simulink model "eme185"  (Simulink 8.6)
settings: Solver=VariableStepAuto  StartTime=0.0  StopTime=10  RelTol=1e-3
values from neighbouring files (symbols this model uses):
  a = [(-2/tau - 1/tau_0) 1/tau 1/tau; 1/tau -2/tau 1/tau; 1/tau 1/tau -2/tau]    [MAE_272A_HW2_Q1a.m]    (also in Vehicle_Dynamic_main.m = 0.624; Vehicle_Dynamic_main_V0.m = 0.624; Vehicle_Dynamic_main_V01.m = 0.624; Vehicle_Dynamic_main_V0605.m = 0.624)
  b = [1/A 0; 0 1/A; 0 0]    [MAE_272A_HW2_Q1a.m]    (also in Vehicle_Dynamic_main.m = 0.624; Vehicle_Dynamic_main_V0.m = 0.624; Vehicle_Dynamic_main_V01.m = 0.624; Vehicle_Dynamic_main_V0605.m = 0.624)
  bL = 60    [simulation_1.m]
  bm = 0.005    [simulation_1.m]
  Ca = 1*0.025    (= 0.025)    [simulation_1.m]
  Cy = 2*20000    (= 40000)    [simulation_1.m]
  gr = 1/20    (= 0.05)    [simulation_1.m]
  initial = [0 0 0 0 (m*g*weight_left/k_spring) (m*g*weight_right/k_spring) ((m*weight_left+mt)*g/k_tire_l) ((m*weight_right+mt)*g/k_tire_r) 0]    [Wegiht_Transfer_Calculator.m]    (also in simulation_1.m = [0 0 0 0 0 0 0 0 0 0])
  Jm = 3.5e-4    (= 0.00035)    [simulation_1.m]
  Jwd = 0.45    [simulation_1.m]
  Jy = 0.4*m*a*b    (= 864)    [master.m]    (also in simulation_1.m = 4250)
  kL = 1400    [simulation_1.m]
  kU = 140    [simulation_1.m]
  l = 0.135    [simulation_1.m]
  m = m_total*weight_front    (= 118.8)    [Wegiht_Transfer_Calculator.m]    (also in master.m = 1600; simulation_1.m = 1800)
  rp = 0.01    [simulation_1.m]
  T = minreal(1-S)    [MAE298_Final_Q2.m]    (also in MAE298_Final_Q22.m = 1-S; MAE298_Final_Q5.m = zpk(minreal(Y*Gp)); MAE_s72A_HW4_Q4.m = 1-S; MAE_s72A_HW4_Q4_5.m = 1-S)
settings Model: Creator=zzLiu  LastModifiedBy=zzLiu
settings DataIOCC: SaveFormat=Dataset  SignalLoggingSaveFormat=Dataset
settings OptimizationCC: ExpressionDepthLimit=128
settings DebuggingCC: UnderspecifiedInitializationDetection=Simplified  MergeDetectMultiDrivingBlocksExec=error  SolverPrmCheckMsg=none  FcnCallInpInsideContextMsg=EnableAllAsError  StateNameClashWarn=none
settings HardwareCC: ProdBitPerPointer=64  ProdLargestAtomicFloat=Float  ProdIntDivRoundTo=Zero  ProdEndianess=LittleEndian  ProdWordSize=64  ProdHWDeviceType=Intel->x86-64 (Windows64)
settings GRTTargetCC: GeneratePreprocessorConditionals=Use local settings  CombineOutputUpdateFcns=on  GRTInterface=off
settings ConfigComp: CovModelRefEnable=off

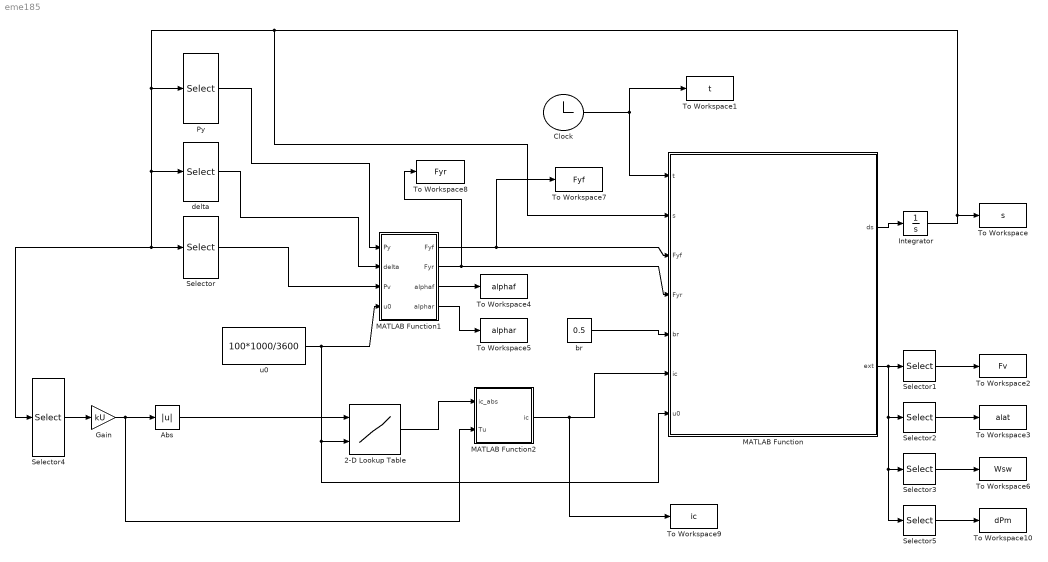
== system eme185 ==
  2-D Lookup Table : Lookup_n-D  BreakpointsForDimension1=[0.0 0.6 1.1 1.6 2.1 2.6 3.2 3.7 4.2 4.7 5.2 5.7 6.3]  BreakpointsForDimension2=[0 5.5556 11.1111 22.2222 27.7778 33.3333]  Table=[0 0 0 1.1 2.0 7.0 14.6 22.3 29.7 37.4 45.0 45.0 45.0;0 0 0 0 0 5.4 12.6 19.1 25.0 31.1 36.5 40.5 40.5;0 0 0 0 0 4.7 10.6 16.4 21.6 27.2 32.4 36.0 36.0;0 0 0 0.5 1.5 4.1 7.7 11.5 15.8 19.8 23.0 23.0 23.0;0 0 0 0 0 2.9 6.1 9.5 12.8 16.7 22.1 22.1 22.1;0 0 0 0 0 2.3 5.0 7.9 11.7 15.1 22.1 22.1 22.1]'  InternalRulePriority=Speed  RndMeth=Simplest  InputSameDT=on
  Abs : Abs
  Clock : Clock
  Gain : Gain  Gain=kU
  Integrator : Integrator  InitialCondition=initial
  MATLAB Function : MATLAB Function  TreatAsAtomicUnit=on
  MATLAB Function1 : MATLAB Function  TreatAsAtomicUnit=on
  MATLAB Function2 : MATLAB Function  TreatAsAtomicUnit=on
  Py : Selector  InputPortWidth=10  IndexOptions=Index vector (dialog)  Indices=[2]  OutputSizes=1
  Selector : Selector  InputPortWidth=10  IndexOptions=Index vector (dialog)  Indices=[1]  OutputSizes=1
  Selector1 : Selector  InputPortWidth=4  IndexOptions=Index vector (dialog)  Indices=[1]  OutputSizes=1
  Selector2 : Selector  InputPortWidth=4  IndexOptions=Index vector (dialog)  Indices=[2]  OutputSizes=1
  Selector3 : Selector  InputPortWidth=4  IndexOptions=Index vector (dialog)  Indices=[3]  OutputSizes=1
  Selector4 : Selector  InputPortWidth=10  IndexOptions=Index vector (dialog)  Indices=[5]  OutputSizes=1
  Selector5 : Selector  InputPortWidth=4  IndexOptions=Index vector (dialog)  Indices=[4]  OutputSizes=1
  To Workspace : ToWorkspace  VariableName=s  SampleTime=-1
  To Workspace1 : ToWorkspace  VariableName=t  SampleTime=-1
  To Workspace10 : ToWorkspace  VariableName=dPm  SaveFormat=Timeseries  SampleTime=-1
  To Workspace2 : ToWorkspace  VariableName=Fv  SaveFormat=Timeseries  SampleTime=-1
  To Workspace3 : ToWorkspace  VariableName=alat  SaveFormat=Timeseries  SampleTime=-1
  To Workspace4 : ToWorkspace  VariableName=alphaf  SaveFormat=Timeseries  SampleTime=-1
  To Workspace5 : ToWorkspace  VariableName=alphar  SaveFormat=Timeseries  SampleTime=-1
  To Workspace6 : ToWorkspace  VariableName=Wsw  SaveFormat=Timeseries  SampleTime=-1
  To Workspace7 : ToWorkspace  VariableName=Fyf  SaveFormat=Timeseries  SampleTime=-1
  To Workspace8 : ToWorkspace  VariableName=Fyr  SaveFormat=Timeseries  SampleTime=-1
  To Workspace9 : ToWorkspace  VariableName=ic  SaveFormat=Timeseries  SampleTime=-1
  br : Constant  Value=0.5
  delta : Selector  InputPortWidth=10  IndexOptions=Index vector (dialog)  Indices=[7]  OutputSizes=1
  u0 : Constant  Value=100*1000/3600
  wires:
  MATLAB Function/1(ds) -> Integrator/1
  Integrator/1 -> MATLAB Function/2(s), Selector/1, Selector4/1, delta/1, Py/1, To Workspace/1
  br/1 -> MATLAB Function/5(br)
  MATLAB Function1/1(Fyf) -> To Workspace7/1, MATLAB Function/3(Fyf)
  MATLAB Function1/2(Fyr) -> MATLAB Function/4(Fyr), To Workspace8/1
  Py/1 -> MATLAB Function1/1(Py)
  delta/1 -> MATLAB Function1/2(delta)
  Clock/1 -> To Workspace1/1, MATLAB Function/1(t)
  u0/1 -> MATLAB Function/7(u0), 2-D Lookup Table/2, MATLAB Function1/4(u0)
  Selector/1 -> MATLAB Function1/3(Pv)
  MATLAB Function1/3(alphaf) -> To Workspace4/1
  MATLAB Function1/4(alphar) -> To Workspace5/1
  MATLAB Function/2(ext) -> Selector5/1, Selector3/1, Selector2/1, Selector1/1
  Selector1/1 -> To Workspace2/1
  Selector2/1 -> To Workspace3/1
  Selector3/1 -> To Workspace6/1
  Selector4/1 -> Gain/1
  Gain/1 -> MATLAB Function2/2(Tu), Abs/1
  Selector5/1 -> To Workspace10/1
  Abs/1 -> 2-D Lookup Table/1
  2-D Lookup Table/1 -> MATLAB Function2/1(ic_abs)
  MATLAB Function2/1(ic) -> To Workspace9/1, MATLAB Function/6(ic)

== matlab function MATLAB Function1 ==
  data: Py input double; Fyf output double; delta input double; a parameter double; b parameter double; Cy parameter double; Jy parameter double; m parameter double; Pv input double; u0 input double; Fyr output double; alphaf output double; alphar output double
function [Fyf,Fyr,alphaf,alphar] = fcn(Py, delta, a, b, Cy,Jy, m, Pv,u0)
%#codegen

wy = Py/Jy;
v = Pv/m;

alphaf = delta - atan((v+a*wy)/u0);
alphar = -atan((v-b*wy)/u0);
Fyf = Cy*alphaf;
Fyr = Cy*alphar;

end

== matlab function MATLAB Function ==
  data: t input double; ds output double; s input double; m parameter double; Jy parameter double; Jwd parameter double; Jm parameter double; a parameter double; b parameter double; l parameter double; Ca parameter double; rp parameter double; gr parameter double; T parameter double; bL parameter double; kL parameter double; kU parameter double; Cy parameter double; Fyf input double; Fyr input double; br input double; ic input double; u0 input double; bm parameter double; ext output double
function [ds,ext] = fcn(t,s,m,Jy,Jwd,Jm,a,b,l,Ca,rp,gr,T,bL,kL,kU,Cy,Fyf,Fyr,br,ic,u0,bm)
%#codegen
% state variables
Pv = s(1);
Py = s(2);
Pwd = s(3);
qL = s(4);
qu = s(5);
Pm = s(6);
delta = s(7);
psi = s(8);
X = s(9);
Y = s(10);

% Angular velocity of steering wheel
steer_angle = 35.122*pi/180;
steer_time = 0.15/0.8;
omega_steer1 = steer_angle/steer_time;
% omega_steer2 = -steer_angle/steer_time;
if t>=1 && t<=1+steer_time
    Wsw = omega_steer1;
% elseif t>=2 && t<2+steer_time
%     Wsw = omega_steer2;
else
    Wsw = 0;
end


dPv = Fyf + Fyr - m/Jy*Py*u0;
dPy = a*Fyf - b*Fyr - l/rp*kL*qL - l*bL/rp*(gr/Jm*Pm - l/rp*(Pwd/Jwd - Py/Jy)) + br*l^2*(Pwd/Jwd - Py/Jy);
dPwd =l/rp*kL*qL + l*bL/rp*(gr/Jm*Pm - l/rp*(Pwd/Jwd - Py/Jy)) - br*l^2*(Pwd/Jwd - Py/Jy) - Ca*Fyf;
dqL = gr*Pm/Jm - l/rp*(Pwd/Jwd - Py/Jy);
dqu = Wsw - gr/Jm*Pm;
dPm = -gr*kL*qL + gr*kU*qu ...
    - gr*bL*(-l/rp*(Pwd/Jwd - Py/Jy) + gr*Pm/Jm) - bm*Pm/Jm...
    + T*ic;
delta_dot = Pwd/Jwd - Py/Jy;

dpsi = Py/Jy;
dX = u0*cos(psi)-Pv/m*sin(psi);
dY = Pv/m*cos(psi) + u0*sin(psi);
alat = dPv/m + u0*Py/Jy;

ds = [dPv dPy dPwd dqL dqu dPm delta_dot dpsi, dX, dY]';
ext = [dPv, alat, Wsw, dPm]';

== matlab function MATLAB Function2 ==
  data: ic_abs input double; ic output double; Tu input double
function ic = fcn(ic_abs,Tu)
%#codegen

if Tu > 0
    ic = ic_abs;
else
    ic = -ic_abs;
end


end
